simulink model "encoder"  (R2015a)
settings: Solver=ode45  StartTime=0.0  StopTime=10.0  RelTol=1e-3
settings Model: Creator=keysie  LastModifiedBy=keysie
settings HardwareCC: TargetBitPerLong=64  TargetBitPerPointer=64  TargetLongLongMode=on  TargetIntDivRoundTo=Zero  TargetEndianess=LittleEndian  TargetWordSize=64  TargetHWDeviceType=MATLAB Host  ProdEqTarget=off
settings RTWCC: SystemTargetFile=rsim.tlc  TemplateMakefile=rsim_default_tmf  Description=Rapid Simulation Target
settings RSimTargetCC: ERTMultiwordTypeDef=System defined  ERTMultiwordLength=256

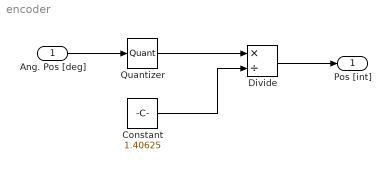
== system encoder ==
  Ang. Pos [deg] : Inport
  Constant : Constant  Value=1.40625
  Divide : Product  Inputs=*/
  Quantizer : Quantizer  QuantizationInterval=1.40625  LinearizeAsGain=off
  Pos [int] : Outport
  wires:
  Ang. Pos [deg]/1 -> Quantizer/1
  Quantizer/1 -> Divide/1
  Divide/1 -> Pos [int]/1
  Constant/1 -> Divide/2
